simulink model "W3P1_model"  (R2020a)
settings: Solver=VariableStepAuto  StartTime=0.0  StopTime=10.0  RelTol=1e-3
settings Model: Creator=avn19  LastModifiedBy=avn19

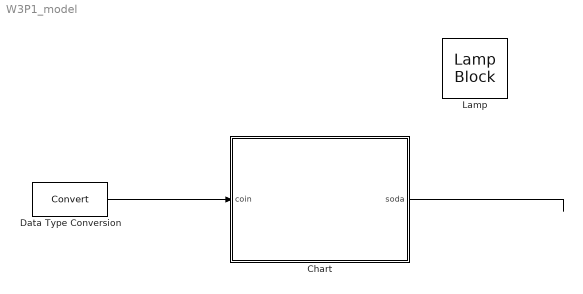
== system W3P1_model ==
  Chart : Stateflow chart  TreatAsAtomicUnit=on
  Data Type Conversion : DataTypeConversion
  Lamp : LampBlock
  wires:
  Data Type Conversion/1 -> Chart/1(coin)
  Chart/1(soda) -> ?

== stateflow chart W3P1_model/Chart ==
  state got_0
  state got_nickel
  state got_dime
  (default) -> got_0
  got_0 -> got_nickel [order 1] : [coin == 1]{soda=0;}
  got_nickel -> got_0 [order 2] : [coin==2]{soda=1;}
  got_dime -> got_0 [order 1] : [coin == 1]{soda = 1;}
  got_0 -> got_dime [order 2] : [coin == 2]{soda = 0;}
  got_nickel -> got_dime [order 1] : [coin == 1]{soda = 0;}
  got_dime -> got_nickel [order 2] : [coin == 2]{soda = 1;}
  data: coin input; soda output
